simulink model "lol_2019"  (R2019a)
settings: Solver=FixedStepAuto  StartTime=0.0  StopTime=5  FixedStep=0.05  MaxStep=0.05  RelTol=1e-3
undefined symbols (not defined in the file or in its folder): Continuous, Time
libraries: simulink x2, ctrlSharedLib x1
settings Model: Creator=alunos_ar  LastModifiedBy=User
settings DebuggingCC: SFMachineParentedDataDiag=error

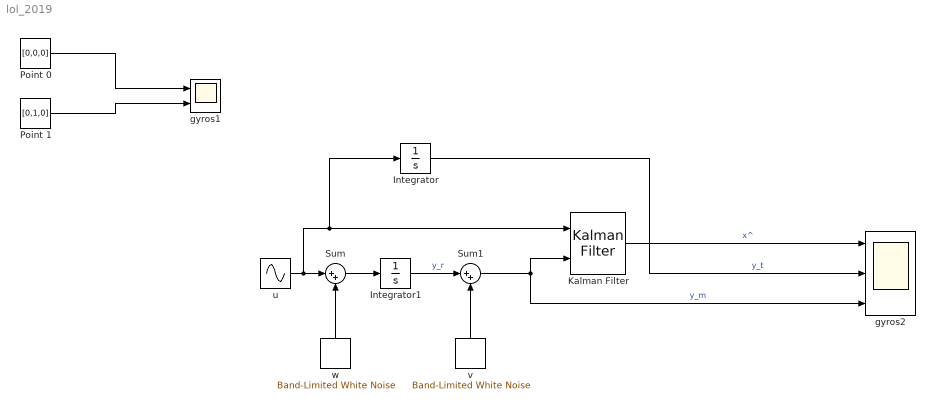
== system lol_2019 ==
  Integrator : Integrator
  Integrator1 : Integrator
  Kalman Filter : ctrlSharedLib/Kalman Filter  TimeDomain=Continuous-Time  UseCurrentEstimator=on  ModelSource=Individual A, B, C, D matrices  ModelSourceVariable=ss(0.95,1,1,0,1)  A=0  B=1  C=1  D=0  NumberOfStates=1  NumberOfInputs=1  NumberOfOutputs=1  InitialEstimateSource=Dialog  X0=0  P0=10  UseK=off  UseGH=off  NumberOfProcessNoiseInputs=1  G=1  TimeInvariantG=on  H=0  TimeInvariantH=on  Q=2  TimeInvariantQ=on  R=1  TimeInvariantR=on  N=0  TimeInvariantN=on  AddInputPort=on  AddEnablePort=off  OutputEstimatedY=off  OutputP=off  Ts=-1
      settings: SourceProductBaseCode=CT
  Point 0 : Constant  Value=[0,0,0]  VectorParams1D=off  SampleTime=-1
  Point 1 : Constant  Value=[0,1,0]
  Sum : Sum  Inputs=|++
  Sum1 : Sum  Inputs=|++
  gyros1 : Scope  NumInputPorts=2
  gyros2 : Scope  NumInputPorts=3
  u : Sin  Amplitude=10  Frequency=10
  v : simulink/Sources/Band-Limited White Noise  Cov=[10^(-2)]  Ts=0.05  seed=[23341]
  w : simulink/Sources/Band-Limited White Noise  Cov=[10^(-2)]  Ts=0.05  seed=[23341]
  wires:
  Point 0/1 -> gyros1/1
  Point 1/1 -> gyros1/2
  Sum/1 -> Integrator1/1
  w/1 -> Sum/2
  Integrator1/1 -> Sum1/1  "y_r"
  Sum1/1 -> gyros2/3, Kalman Filter/2  "y_m"
  v/1 -> Sum1/2
  Kalman Filter/1 -> gyros2/1  "x^"
  Integrator/1 -> gyros2/2  "y_t"
  u/1 -> Integrator/1, Kalman Filter/1, Sum/1
